simulink model "Model_Simulink"  (Simulink 8.7)
settings: Solver=ode3  StartTime=0.0  StopTime=50  FixedStep=0.0001  RelTol=1e-3
values from neighbouring files (symbols this model uses):
  A = 40    [Courbe2d.m]    (also in Donneesp2.m; main.m)
  c = 200000    [Donneesp2.m]
  k = 400000    [Courbe2d.m]    (also in Donneesp2.m; main.m = 10000000)
  m = 25    [Donneesp2.m]
  v0 = 0    [Donneesp2.m]    (also in main.m)
  w = 50    [Donneesp2.m]    (also in main.m = Wn)
  x0 = 0    [Donneesp2.m]    (also in main.m)
settings Model: Creator=p202400  LastModifiedBy=sitanb
settings DataIOCC: SignalLoggingSaveFormat=ModelDataLogs
settings OptimizationCC: ExpressionDepthLimit=2147483647
settings DebuggingCC: SolverPrmCheckMsg=warning  FcnCallInpInsideContextMsg=UseLocalSettings  StateNameClashWarn=warning
settings GRTTargetCC: CombineOutputUpdateFcns=off  GRTInterface=on

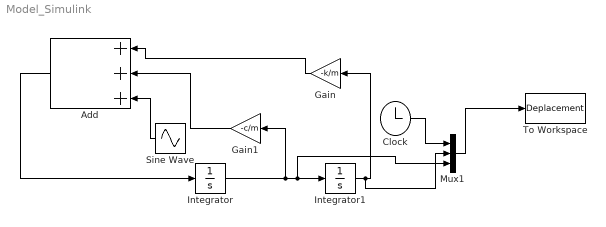
== system Model_Simulink ==
  Add : Sum  Inputs=+++
  Clock : Clock
  Gain : Gain  Gain=-k/m
  Gain1 : Gain  Gain=-c/m
  Integrator : Integrator  InitialCondition=v0
  Integrator1 : Integrator  InitialCondition=x0
  Mux1 : Mux  Inputs=3
  Sine Wave : Sin  Amplitude=A/m  Frequency=w  SampleTime=0
  To Workspace : ToWorkspace  VariableName=Deplacement  SampleTime=-1
  wires:
  Integrator/1 -> Mux1/3, Integrator1/1, Gain1/1
  Integrator1/1 -> Gain/1, Mux1/2
  Gain1/1 -> Add/2
  Gain/1 -> Add/1
  Add/1 -> Integrator/1
  Clock/1 -> Mux1/1
  Mux1/1 -> To Workspace/1
  Sine Wave/1 -> Add/3
